simulink model "Control_BC"  (R2023b)
settings: Solver=VariableStepAuto  StartTime=0.0  StopTime=10  RelTol=1e-3
settings Model: Creator=ricfe  LastModifiedBy=ricfe

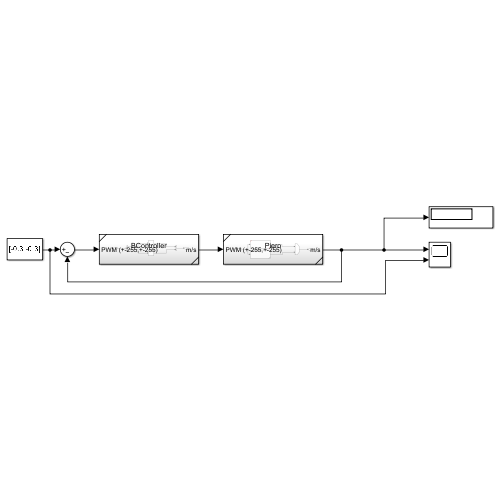
[thumbnail: Simulink's stored preview of the top-level diagram]
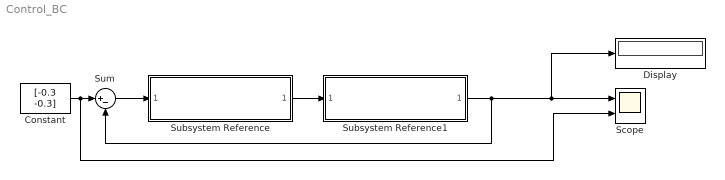
== system Control_BC ==
  Constant : Constant  Value=[-0.3 -0.3]
  Display : Display
  Scope : Scope  NumInputPorts=2
  Subsystem Reference : Subsystem  ReferencedSubsystem=BController
  Subsystem Reference1 : Subsystem  ReferencedSubsystem=Piero
  Sum : Sum  Inputs=|+-
  wires:
  Subsystem Reference1/1 -> Sum/2, Display/1, Scope/1
  Constant/1 -> Scope/2, Sum/1
  Subsystem Reference/1 -> Subsystem Reference1/1
  Sum/1 -> Subsystem Reference/1
